simulink model "saveDataToFile"  (R2019b)
settings: Solver=FixedStepDiscrete  StartTime=0.0  StopTime=Inf  FixedStep=sampleTime  RelTol=1e-3  EnableMultiTasking=on
InitFcn:
  | sampleTime = 1/200;
libraries: xpcrtudplib x1, xpcutilitieslib x1
settings Model: EnablePacing=on  Creator=student  LastModifiedBy=student
settings DataIOCC: LimitDataPoints=on  SaveFormat=Array  ReturnWorkspaceOutputs=off
settings OptimizationCC: LifeSpan=inf
settings DebuggingCC: UnderspecifiedInitializationDetection=Classic  MergeDetectMultiDrivingBlocksExec=none  SolverPrmCheckMsg=warning  StateNameClashWarn=warning  SFUnexpectedBacktrackingDiag=warning  SFNoUnconditionalDefaultTransitionDiag=warning  SFExecutionAtInitializationDiag=none  ArithmeticOperatorsInVariantConditions=warning
settings HardwareCC: ProdBitPerPointer=32  ProdBitPerSizeT=32  ProdBitPerPtrDiffT=32  ProdLargestAtomicFloat=None  ProdIntDivRoundTo=Undefined  ProdEndianess=Unspecified  ProdWordSize=32  ProdHWDeviceType=32-bit Generic
settings ModelReferenceCC: PropagateSignalLabelsOutOfModel=off
settings SFSimCC: SimUseLocalCustomCode=off  CustomCodeUndefinedFunction=UseInterfaceOnly
settings RTWCC: RTWUseLocalCustomCode=off
settings CodeAppCC: StateflowObjectComments=on
settings GRTTargetCC: TargetLangStandard=C89/C90 (ANSI)  GeneratePreprocessorConditionals=Disable all
settings ConfigComp: CovMetricSettings=dw  CovHtmlReporting=on  CovSaveCumulativeToWorkspaceVar=on  CovSaveSingleToWorkspaceVar=on  CovExternalEMLEnable=off

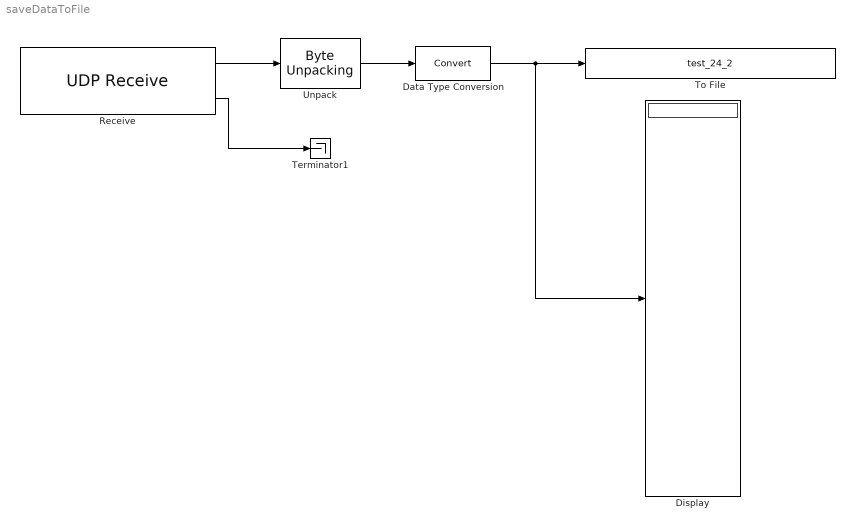
== system saveDataToFile ==
  Data Type Conversion : DataTypeConversion  SampleTime=sampleTime
  Display : Display
  Receive : xpcrtudplib/UDP Receive  ipAddressVal=Use host-target connection  localPort=25010  rcvWidth=4*117  rcvFmAny=off  fmAddress=192.168.65.245  rcvMulticast=off  multicastAddress={}  maxUDPQueue=8  sampleTime=sampleTime
      settings: SourceProductName=Simulink Real-Time
  Terminator1 : Terminator
  To File : ToFile  Filename=test_24_2  MatrixName=data  SampleTime=sampleTime
  Unpack : xpcutilitieslib/Byte Unpacking   MaskUnpackedDataTypes={'single'}  MaskUnpackedDataSizes={[117]}  MaskAlignment=1
      settings: SourceProductName=Simulink Real-Time  SourceProductBaseCode=XP
  wires:
  Receive/1 -> Unpack/1
  Unpack/1 -> Data Type Conversion/1
  Receive/2 -> Terminator1/1
  Data Type Conversion/1 -> Display/1, To File/1
